simulink model "GenFaultyData"  (R2014a)
settings: Solver=FixedStepDiscrete  StartTime=0.0  StopTime=SimLength  FixedStep=SampleTime  RelTol=1e-3
settings Model: Creator=georg  LastModifiedBy=Maik
settings DataIOCC: SaveOutput=off  SaveTime=off

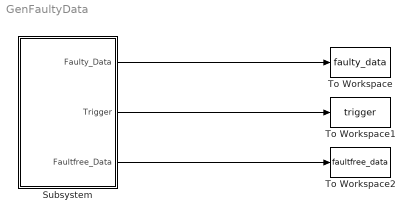
== system GenFaultyData ==
  Subsystem : Subsystem
  To Workspace : ToWorkspace  VariableName=faulty_data  SaveFormat=Timeseries  SampleTime=-1
  To Workspace1 : ToWorkspace  VariableName=trigger  SaveFormat=Timeseries  SampleTime=-1
  To Workspace2 : ToWorkspace  VariableName=faultfree_data  SaveFormat=Timeseries  SampleTime=-1
  wires:
  Subsystem/1(Faulty_Data) -> To Workspace/1
  Subsystem/2(Trigger) -> To Workspace1/1
  Subsystem/3(Faultfree_Data) -> To Workspace2/1

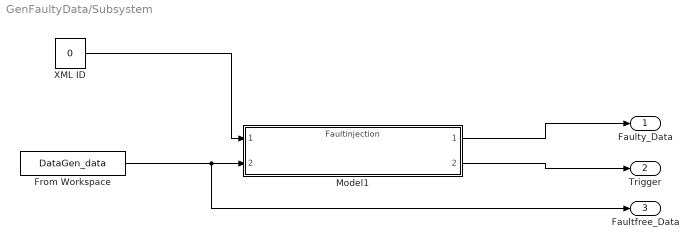
== system GenFaultyData/Subsystem ==
  From Workspace : FromWorkspace  VariableName=DataGen_data  SampleTime=0
  Model1 : ModelReference  ModelNameDialog=Faultinjection.slx  SimulationMode=Normal  ModelReferenceVersion=1.10  CopyOfModelName=Faultinjection.slx  DefaultDataLogging=on
  XML ID : Constant  Value=0  OutDataTypeStr=single
  Faulty_Data : Outport
  Trigger : Outport  Port=2  OutDataTypeStr=Bus: TriggerBus
  Faultfree_Data : Outport  Port=3
  wires:
  From Workspace/1 -> Faultfree_Data/1, Model1/2
  Model1/1 -> Faulty_Data/1
  XML ID/1 -> Model1/1
  Model1/2 -> Trigger/1
